simulink model "ABS_Bosch_09st"  (R2023a)
settings: Solver=ode45  StartTime=0  StopTime=20  FixedStep=0.001  RelTol=1e-3  AbsTol=1e-6
undefined symbols (not defined in the file or in its folder): DiscIntNeverNeededParam
libraries: simulink x18, dspsigops x4, Solver_SF x1
settings Model: ExtModeTrigMode=oneshot  Creator=jhu  LastModifiedBy=USER
settings SolverCC: AutoScaleAbsTol=off  AlgebraicLoopSolver=TrustRegion
settings DataIOCC: SaveFormat=Array  SignalLoggingSaveFormat=ModelDataLogs  ReturnWorkspaceOutputs=off  SignalLoggingName=sigsOut
settings OptimizationCC: BlockReduction=off  BooleanDataType=off  ExpressionDepthLimit=2147483647  LifeSpan=inf
settings DebuggingCC: SaveWithParameterizedLinksMsg=none  UnderspecifiedInitializationDetection=Classic  MergeDetectMultiDrivingBlocksExec=none  SignalResolutionControl=TryResolveAllWithWarning  MultiTaskDSMMsg=warning  MultiTaskCondExecSysMsg=none  FcnCallInpInsideContextMsg=warning  UnconnectedInputMsg=warning  UnconnectedOutputMsg=warning  UnconnectedLineMsg=warning  StateNameClashWarn=warning  SFUnexpectedBacktrackingDiag=warning  SFNoUnconditionalDefaultTransitionDiag=warning  SFExecutionAtInitializationDiag=none  ArithmeticOperatorsInVariantConditions=warning
settings HardwareCC: ProdBitPerPointer=32  ProdBitPerSizeT=32  ProdBitPerPtrDiffT=32  ProdLargestAtomicFloat=None  ProdIntDivRoundTo=Undefined  ProdEndianess=Unspecified  ProdWordSize=32  ProdHWDeviceType=32-bit Generic  TargetUnknown=on
settings ModelReferenceCC: PropagateSignalLabelsOutOfModel=off
settings SFSimCC: SimUseLocalCustomCode=off  CustomCodeUndefinedFunction=UseInterfaceOnly
settings RTWCC: TemplateMakefile=grt_vc.tmf  RTWUseLocalCustomCode=off
settings CodeAppCC: StateflowObjectComments=on
settings GRTTargetCC: TargetFcnLib=ansi_tfl_tmw.mat  TargetLangStandard=C89/C90 (ANSI)  CombineOutputUpdateFcns=off  GRTInterface=on
settings ConfigComp: CovMetricSettings=dw  CovSaveCumulativeToWorkspaceVar=on  CovSaveSingleToWorkspaceVar=on  CovExternalEMLEnable=off

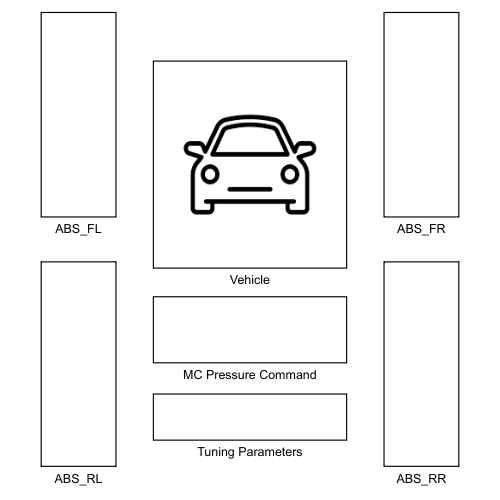
[thumbnail: Simulink's stored preview of the top-level diagram]
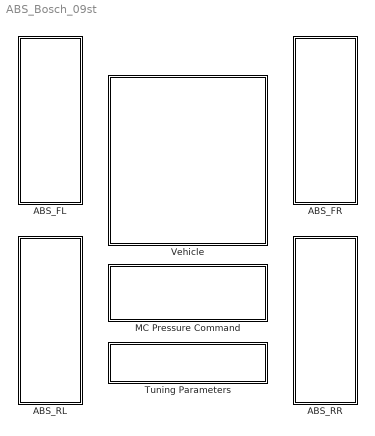
== system ABS_Bosch_09st ==
  ABS_FL : Subsystem
  ABS_FR : Subsystem
  ABS_RL : Subsystem
  ABS_RR : Subsystem
  MC Pressure Command : Subsystem
  Tuning Parameters : Subsystem
  Vehicle : Subsystem
      mask Display: image('C:\Users\USER\Downloads\vehicle_icon.png'); % Use "Edit Image" on toolstrip to change.

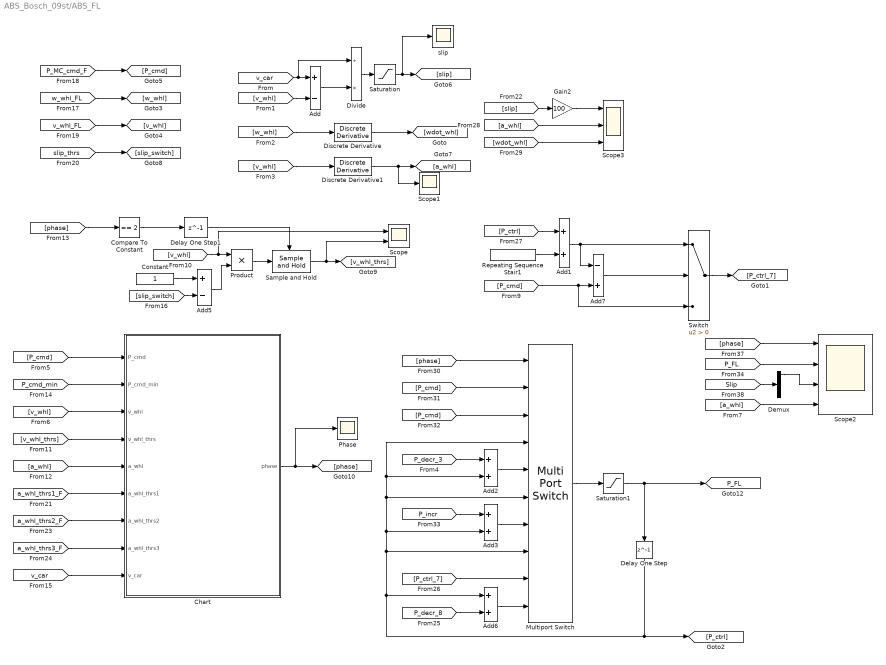
== system ABS_Bosch_09st/ABS_FL ==
  Add : Sum  Inputs=+-
  Add{1..3,6} (4 alike) : Sum
  Add5 : Sum  Inputs=+-
  Add7 : Sum  Inputs=-+
  Chart : Stateflow chart  TreatAsAtomicUnit=on
      settings: PortSchema="{\"entries\":[{\"content\":{\"sides\":[{\"content\":{\"connectorIds\":[\"In4\",\"In5\",\"In2\",\"In9\",\"In1\",\"In6\",\"In7\",\"In8\",\"In3\"]},\"type\":\"ConnectorPlacement.EquallySpacedRectSide\",\"uuid\":\"d1b40d47-5080-4bdb-9b64-2db0b8a6d570\"},{\"content\":{\"connectorIds\":[\"Out1\"],\"side\":\"RIGHT\"},\"type\":\"ConnectorPlacement.EquallySpacedRectSide\",\"uuid\":\"3562d231-244b-4945-a90c-51a654d62f0f\"},{\"content\":{\"side\":\"TOP\"},\"type\":\"ConnectorPlacement.EquallySpacedRectSide\",\"uuid\":\"6c914ffe-04dc-4ab2-bade-76d69248353c\"}]},\"type\":\"ConnectorPlacement.EquallySpacedConnector\",\"uuid\":\"36a59ec9-6bc3-461d-a020-c1da85e3b47f\"}],\"packageUris\":[\"http://schema.mathworks.com/mf0/Connector/R2020b\"],\"version\":\"1.0\"}"
  Compare To Constant : simulink/Logic and Bit Operations/Compare To Constant  relop===  const=2  OutDataTypeStr=boolean
  Constant : Constant
  Delay One Step : Delay  DelayLength=1  SampleTime=0.01
  Delay One Step1 : Delay  DelayLength=1  SampleTime=0.01
  Demux : Demux
  Discrete Derivative : simulink/Discrete/Discrete Derivative  gainval=1.0  ICPrevScaledInput=0.0  OutMin=[]  OutMax=[]  OutDataType=fixdt(1, 16)  OutScaling=2^-10  DoSatur=off
  Discrete Derivative1 : simulink/Discrete/Discrete Derivative  gainval=1.0  ICPrevScaledInput=0.0  OutMin=[]  OutMax=[]  OutDataType=fixdt(1, 16)  OutScaling=2^-10  DoSatur=off
  Divide : Product  Inputs=/*
  Gain2 : Gain  Gain=100
  Multiport Switch : MultiPortSwitch  DataPortOrder=Zero-based contiguous  Inputs=9  zeroidx=on  SaturateOnIntegerOverflow=off  InputSameDT=off
  Phase : Scope
  Product : Product
  Repeating Sequence Stair1 : simulink/Sources/Repeating Sequence Stair  OutValues=[0.2 0].'  tsamp=0.01  OutMin=[]  OutMax=[]  OutDataTypeStr=double  OutputDataTypeScalingMode=double  OutDataType=fixdt(0,8)  ConRadixGroup=Best Precision: Vector-wise  OutScaling=2^-12
  Sample and Hold : dspsigops/Sample and Hold  trig=Rising edge  initCond=0  latchinput=off
  Saturation : Saturate  UpperLimit=1  LowerLimit=-1
  Saturation1 : Saturate  UpperLimit=6  LowerLimit=0
  Scope : Scope  NumInputPorts=2
  Scope1 : Scope
  Scope2 : Scope  NumInputPorts=4
  Scope3 : Scope  NumInputPorts=3
  Switch : Switch  Criteria=u2 > Threshold  SaturateOnIntegerOverflow=off  InputSameDT=off
  slip : Scope
  tag scope: P_FL=global
  wires:
  Delay One Step/1 -> [P_ctrl], Add6/1, Multiport Switch/6, Add2/2, Multiport Switch/4, Add3/2, Multiport Switch/8
  Switch/1 -> [P_ctrl_7]
  Add7/1 -> Switch/2
  [P_cmd] -> Add7/2, Switch/3
  Add1/1 -> Add7/1, Switch/1
  Repeating Sequence Stair1/1 -> Add1/2
  [P_ctrl] -> Add1/1
  [v_car] -> Divide/1, Add/1
  [v_whl] -> Add/2
  Add/1 -> Divide/2
  Divide/1 -> Saturation/1
  Saturation/1 -> slip/1, [slip]
  [w_whl] -> Discrete Derivative/1
  Discrete Derivative/1 -> [wdot_whl]
  [v_whl] -> Discrete Derivative1/1
  Discrete Derivative1/1 -> Scope1/1, [a_whl]
  [slip_thrs] -> [slip_switch]
  [v_whl] -> Scope/1, Product/1
  Sample and Hold/1 -> Scope/2, [v_whl_thrs]
  Chart/1(phase) -> Phase/1, [phase]
  [w_whl_FL] -> [w_whl]
  [v_whl_FL] -> [v_whl]
  [P_MC_cmd_F] -> [P_cmd]
  [slip] -> Gain2/1
  [a_whl] -> Scope3/2
  [wdot_whl] -> Scope3/3
  Gain2/1 -> Scope3/1
  [phase] -> Multiport Switch/1
  [P_cmd] -> Multiport Switch/2
  [P_cmd] -> Multiport Switch/3
  Multiport Switch/1 -> Saturation1/1
  Add2/1 -> Multiport Switch/5
  [P_decr_3] -> Add2/1
  Add3/1 -> Multiport Switch/7
  [P_ctrl_7] -> Multiport Switch/9
  Saturation1/1 -> Delay One Step/1, [P_FL]
  [P_incr] -> Add3/1
  Constant/1 -> Add5/1
  [slip_switch] -> Add5/2
  Add5/1 -> Product/2
  Product/1 -> Sample and Hold/1
  [phase] -> Scope2/1
  [P_FL] -> Scope2/2
  [P_cmd] -> Chart/4(P_cmd)
  [P_cmd_min] -> Chart/5(P_cmd_min)
  [v_whl] -> Chart/2(v_whl)
  [v_whl_thrs] -> Chart/9(v_whl_thrs)
  [a_whl] -> Chart/1(a_whl)
  [v_car] -> Chart/3(v_car)
  [a_whl] -> Scope2/4
  [phase] -> Compare To Constant/1
  Compare To Constant/1 -> Delay One Step1/1
  Delay One Step1/1 -> Sample and Hold/Trigger
  [a_whl_thrs1_F] -> Chart/6(a_whl_thrs1)
  [a_whl_thrs2_F] -> Chart/7(a_whl_thrs2)
  [a_whl_thrs3_F] -> Chart/8(a_whl_thrs3)
  Add6/1 -> Multiport Switch/10
  [P_decr_8] -> Add6/2
  [Slip] -> Demux/1
  Demux/1 -> Scope2/3

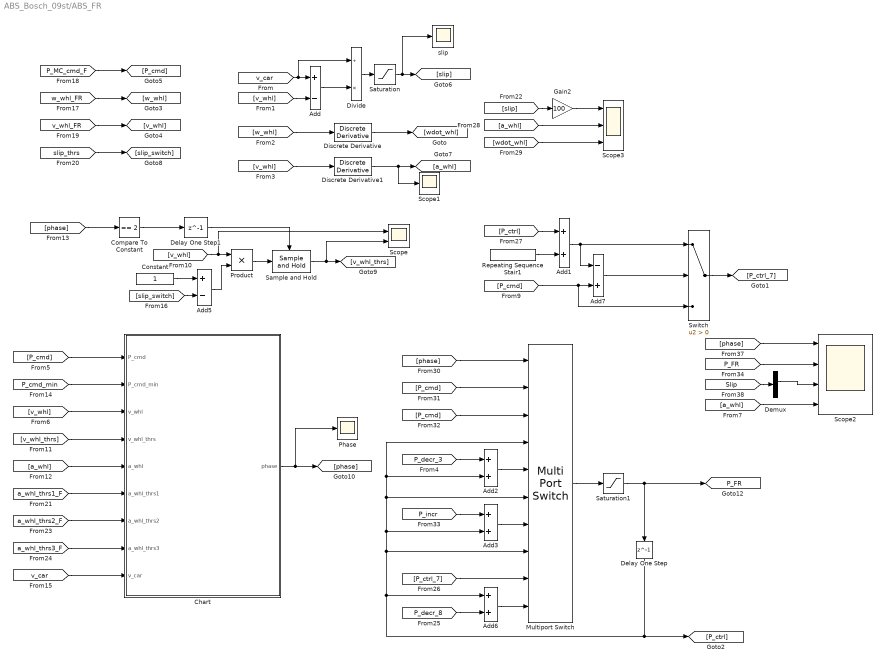
== system ABS_Bosch_09st/ABS_FR ==
  Add : Sum  Inputs=+-
  Add{1..3,6} (4 alike) : Sum
  Add5 : Sum  Inputs=+-
  Add7 : Sum  Inputs=-+
  Chart : Stateflow chart  TreatAsAtomicUnit=on
      settings: PortSchema="{\"entries\":[{\"content\":{\"sides\":[{\"content\":{\"connectorIds\":[\"In4\",\"In5\",\"In2\",\"In9\",\"In1\",\"In6\",\"In7\",\"In8\",\"In3\"]},\"type\":\"ConnectorPlacement.EquallySpacedRectSide\",\"uuid\":\"d1b40d47-5080-4bdb-9b64-2db0b8a6d570\"},{\"content\":{\"connectorIds\":[\"Out1\"],\"side\":\"RIGHT\"},\"type\":\"ConnectorPlacement.EquallySpacedRectSide\",\"uuid\":\"3562d231-244b-4945-a90c-51a654d62f0f\"},{\"content\":{\"side\":\"TOP\"},\"type\":\"ConnectorPlacement.EquallySpacedRectSide\",\"uuid\":\"6c914ffe-04dc-4ab2-bade-76d69248353c\"}]},\"type\":\"ConnectorPlacement.EquallySpacedConnector\",\"uuid\":\"36a59ec9-6bc3-461d-a020-c1da85e3b47f\"}],\"packageUris\":[\"http://schema.mathworks.com/mf0/Connector/R2020b\"],\"version\":\"1.0\"}"
  Compare To Constant : simulink/Logic and Bit Operations/Compare To Constant  relop===  const=2  OutDataTypeStr=boolean
  Constant : Constant
  Delay One Step : Delay  DelayLength=1  SampleTime=0.01
  Delay One Step1 : Delay  DelayLength=1  SampleTime=0.01
  Demux : Demux
  Discrete Derivative : simulink/Discrete/Discrete Derivative  gainval=1.0  ICPrevScaledInput=0.0  OutMin=[]  OutMax=[]  OutDataType=fixdt(1, 16)  OutScaling=2^-10  DoSatur=off
  Discrete Derivative1 : simulink/Discrete/Discrete Derivative  gainval=1.0  ICPrevScaledInput=0.0  OutMin=[]  OutMax=[]  OutDataType=fixdt(1, 16)  OutScaling=2^-10  DoSatur=off
  Divide : Product  Inputs=/*
  Gain2 : Gain  Gain=100
  Multiport Switch : MultiPortSwitch  DataPortOrder=Zero-based contiguous  Inputs=9  zeroidx=on  SaturateOnIntegerOverflow=off  InputSameDT=off
  Phase : Scope
  Product : Product
  Repeating Sequence Stair1 : simulink/Sources/Repeating Sequence Stair  OutValues=[0.2 0].'  tsamp=0.01  OutMin=[]  OutMax=[]  OutDataTypeStr=double  OutputDataTypeScalingMode=double  OutDataType=fixdt(0,8)  ConRadixGroup=Best Precision: Vector-wise  OutScaling=2^-12
  Sample and Hold : dspsigops/Sample and Hold  trig=Rising edge  initCond=0  latchinput=off
  Saturation : Saturate  UpperLimit=1  LowerLimit=-1
  Saturation1 : Saturate  UpperLimit=6  LowerLimit=0
  Scope : Scope  NumInputPorts=2
  Scope1 : Scope
  Scope2 : Scope  NumInputPorts=4
  Scope3 : Scope  NumInputPorts=3
  Switch : Switch  Criteria=u2 > Threshold  SaturateOnIntegerOverflow=off  InputSameDT=off
  slip : Scope
  tag scope: P_FR=global
  wires:
  [P_decr_8] -> Add6/2
  Add6/1 -> Multiport Switch/10
  [a_whl_thrs3_F] -> Chart/8(a_whl_thrs3)
  [a_whl_thrs2_F] -> Chart/7(a_whl_thrs2)
  [a_whl_thrs1_F] -> Chart/6(a_whl_thrs1)
  Delay One Step1/1 -> Sample and Hold/Trigger
  Compare To Constant/1 -> Delay One Step1/1
  [phase] -> Compare To Constant/1
  [a_whl] -> Scope2/4
  [v_car] -> Chart/3(v_car)
  [a_whl] -> Chart/1(a_whl)
  [v_whl_thrs] -> Chart/9(v_whl_thrs)
  [v_whl] -> Chart/2(v_whl)
  [P_cmd_min] -> Chart/5(P_cmd_min)
  [P_cmd] -> Chart/4(P_cmd)
  [Slip] -> Demux/1
  [P_FR] -> Scope2/2
  [phase] -> Scope2/1
  Product/1 -> Sample and Hold/1
  Add5/1 -> Product/2
  [slip_switch] -> Add5/2
  Constant/1 -> Add5/1
  [P_incr] -> Add3/1
  Saturation1/1 -> [P_FR], Delay One Step/1
  [P_ctrl_7] -> Multiport Switch/9
  Add3/1 -> Multiport Switch/7
  [P_decr_3] -> Add2/1
  Add2/1 -> Multiport Switch/5
  Multiport Switch/1 -> Saturation1/1
  [P_cmd] -> Multiport Switch/3
  [P_cmd] -> Multiport Switch/2
  [phase] -> Multiport Switch/1
  Gain2/1 -> Scope3/1
  [wdot_whl] -> Scope3/3
  [a_whl] -> Scope3/2
  [slip] -> Gain2/1
  [P_MC_cmd_F] -> [P_cmd]
  [v_whl_FR] -> [v_whl]
  [w_whl_FR] -> [w_whl]
  Chart/1(phase) -> [phase], Phase/1
  Sample and Hold/1 -> [v_whl_thrs], Scope/2
  [v_whl] -> Product/1, Scope/1
  [slip_thrs] -> [slip_switch]
  Discrete Derivative1/1 -> [a_whl], Scope1/1
  [v_whl] -> Discrete Derivative1/1
  Discrete Derivative/1 -> [wdot_whl]
  [w_whl] -> Discrete Derivative/1
  Saturation/1 -> [slip], slip/1
  Divide/1 -> Saturation/1
  Add/1 -> Divide/2
  [v_whl] -> Add/2
  [v_car] -> Add/1, Divide/1
  [P_ctrl] -> Add1/1
  Repeating Sequence Stair1/1 -> Add1/2
  Add1/1 -> Switch/1, Add7/1
  [P_cmd] -> Switch/3, Add7/2
  Add7/1 -> Switch/2
  Switch/1 -> [P_ctrl_7]
  Delay One Step/1 -> Multiport Switch/8, Add3/2, Multiport Switch/6, Multiport Switch/4, Add2/2, Add6/1, [P_ctrl]
  Demux/2 -> Scope2/3

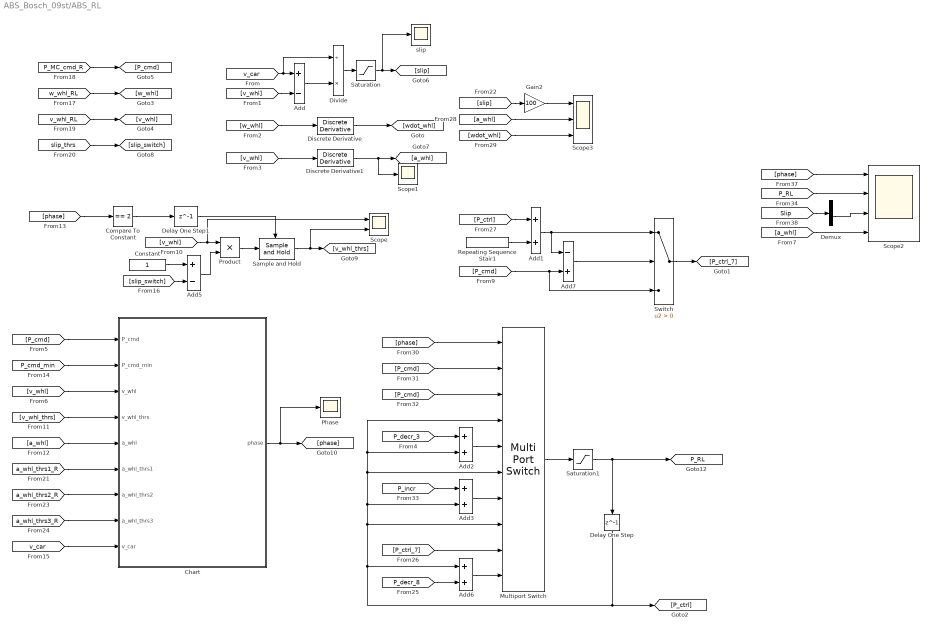
== system ABS_Bosch_09st/ABS_RL ==
  Add : Sum  Inputs=+-
  Add{1..3,6} (4 alike) : Sum
  Add5 : Sum  Inputs=+-
  Add7 : Sum  Inputs=-+
  Chart : Stateflow chart  TreatAsAtomicUnit=on
      settings: PortSchema="{\"entries\":[{\"content\":{\"sides\":[{\"content\":{\"connectorIds\":[\"In4\",\"In5\",\"In2\",\"In9\",\"In1\",\"In6\",\"In7\",\"In8\",\"In3\"]},\"type\":\"ConnectorPlacement.EquallySpacedRectSide\",\"uuid\":\"d1b40d47-5080-4bdb-9b64-2db0b8a6d570\"},{\"content\":{\"connectorIds\":[\"Out1\"],\"side\":\"RIGHT\"},\"type\":\"ConnectorPlacement.EquallySpacedRectSide\",\"uuid\":\"3562d231-244b-4945-a90c-51a654d62f0f\"},{\"content\":{\"side\":\"TOP\"},\"type\":\"ConnectorPlacement.EquallySpacedRectSide\",\"uuid\":\"6c914ffe-04dc-4ab2-bade-76d69248353c\"}]},\"type\":\"ConnectorPlacement.EquallySpacedConnector\",\"uuid\":\"36a59ec9-6bc3-461d-a020-c1da85e3b47f\"}],\"packageUris\":[\"http://schema.mathworks.com/mf0/Connector/R2020b\"],\"version\":\"1.0\"}"
  Compare To Constant : simulink/Logic and Bit Operations/Compare To Constant  relop===  const=2  OutDataTypeStr=boolean
  Constant : Constant
  Delay One Step : Delay  DelayLength=1  SampleTime=0.01
  Delay One Step1 : Delay  DelayLength=1  SampleTime=0.01
  Demux : Demux
  Discrete Derivative : simulink/Discrete/Discrete Derivative  gainval=1.0  ICPrevScaledInput=0.0  OutMin=[]  OutMax=[]  OutDataType=fixdt(1, 16)  OutScaling=2^-10  DoSatur=off
  Discrete Derivative1 : simulink/Discrete/Discrete Derivative  gainval=1.0  ICPrevScaledInput=0.0  OutMin=[]  OutMax=[]  OutDataType=fixdt(1, 16)  OutScaling=2^-10  DoSatur=off
  Divide : Product  Inputs=/*
  Gain2 : Gain  Gain=100
  Multiport Switch : MultiPortSwitch  DataPortOrder=Zero-based contiguous  Inputs=9  zeroidx=on  SaturateOnIntegerOverflow=off  InputSameDT=off
  Phase : Scope
  Product : Product
  Repeating Sequence Stair1 : simulink/Sources/Repeating Sequence Stair  OutValues=[0.2 0].'  tsamp=0.01  OutMin=[]  OutMax=[]  OutDataTypeStr=double  OutputDataTypeScalingMode=double  OutDataType=fixdt(0,8)  ConRadixGroup=Best Precision: Vector-wise  OutScaling=2^-12
  Sample and Hold : dspsigops/Sample and Hold  trig=Rising edge  initCond=0  latchinput=off
  Saturation : Saturate  UpperLimit=1  LowerLimit=-1
  Saturation1 : Saturate  UpperLimit=5  LowerLimit=0
  Scope : Scope  NumInputPorts=2
  Scope1 : Scope
  Scope2 : Scope  NumInputPorts=4
  Scope3 : Scope  NumInputPorts=3
  Switch : Switch  Criteria=u2 > Threshold  SaturateOnIntegerOverflow=off  InputSameDT=off
  slip : Scope
  tag scope: P_RL=global
  wires:
  Delay One Step/1 -> [P_ctrl], Add6/1, Multiport Switch/6, Add2/2, Multiport Switch/4, Add3/2, Multiport Switch/8
  Switch/1 -> [P_ctrl_7]
  Add7/1 -> Switch/2
  [P_cmd] -> Add7/2, Switch/3
  Add1/1 -> Add7/1, Switch/1
  Repeating Sequence Stair1/1 -> Add1/2
  [P_ctrl] -> Add1/1
  [v_car] -> Divide/1, Add/1
  [v_whl] -> Add/2
  Add/1 -> Divide/2
  Divide/1 -> Saturation/1
  Saturation/1 -> slip/1, [slip]
  [w_whl] -> Discrete Derivative/1
  Discrete Derivative/1 -> [wdot_whl]
  [v_whl] -> Discrete Derivative1/1
  Discrete Derivative1/1 -> Scope1/1, [a_whl]
  [slip_thrs] -> [slip_switch]
  [v_whl] -> Scope/1, Product/1
  Sample and Hold/1 -> Scope/2, [v_whl_thrs]
  Chart/1(phase) -> Phase/1, [phase]
  [w_whl_RL] -> [w_whl]
  [v_whl_RL] -> [v_whl]
  [P_MC_cmd_R] -> [P_cmd]
  [slip] -> Gain2/1
  [a_whl] -> Scope3/2
  [wdot_whl] -> Scope3/3
  Gain2/1 -> Scope3/1
  [phase] -> Multiport Switch/1
  [P_cmd] -> Multiport Switch/2
  [P_cmd] -> Multiport Switch/3
  Multiport Switch/1 -> Saturation1/1
  Add2/1 -> Multiport Switch/5
  [P_decr_3] -> Add2/1
  Add3/1 -> Multiport Switch/7
  [P_ctrl_7] -> Multiport Switch/9
  Saturation1/1 -> Delay One Step/1, [P_RL]
  [P_incr] -> Add3/1
  Constant/1 -> Add5/1
  [slip_switch] -> Add5/2
  Add5/1 -> Product/2
  Product/1 -> Sample and Hold/1
  [phase] -> Scope2/1
  [P_RL] -> Scope2/2
  [P_cmd] -> Chart/4(P_cmd)
  [P_cmd_min] -> Chart/5(P_cmd_min)
  [v_whl] -> Chart/2(v_whl)
  [v_whl_thrs] -> Chart/9(v_whl_thrs)
  [a_whl] -> Chart/1(a_whl)
  [v_car] -> Chart/3(v_car)
  [a_whl] -> Scope2/4
  [phase] -> Compare To Constant/1
  Compare To Constant/1 -> Delay One Step1/1
  Delay One Step1/1 -> Sample and Hold/Trigger
  [a_whl_thrs1_R] -> Chart/6(a_whl_thrs1)
  [a_whl_thrs2_R] -> Chart/7(a_whl_thrs2)
  [a_whl_thrs3_R] -> Chart/8(a_whl_thrs3)
  Add6/1 -> Multiport Switch/10
  [P_decr_8] -> Add6/2
  [Slip] -> Demux/1
  Demux/3 -> Scope2/3

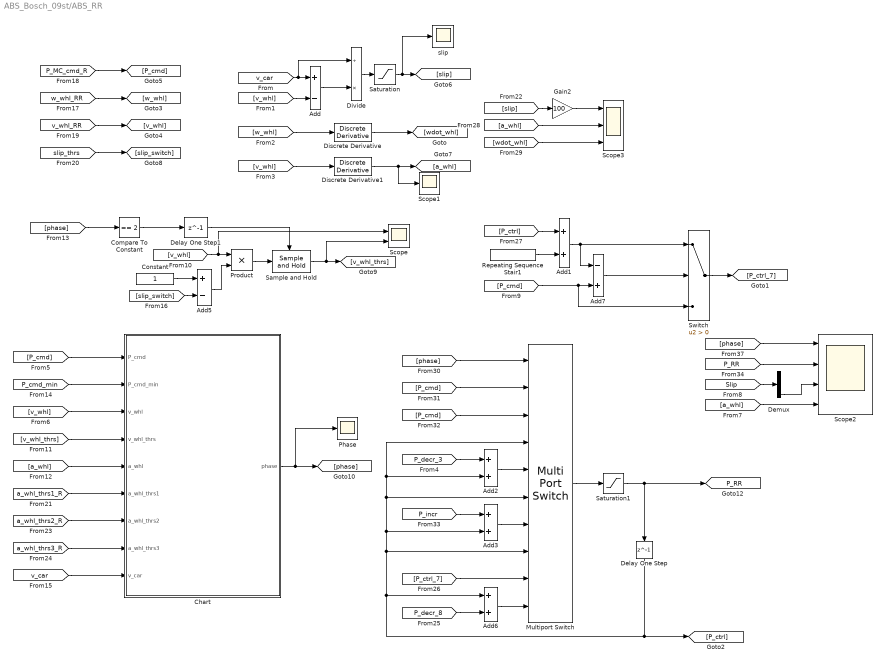
== system ABS_Bosch_09st/ABS_RR ==
  Add : Sum  Inputs=+-
  Add{1..3,6} (4 alike) : Sum
  Add5 : Sum  Inputs=+-
  Add7 : Sum  Inputs=-+
  Chart : Stateflow chart  TreatAsAtomicUnit=on
      settings: PortSchema="{\"entries\":[{\"content\":{\"sides\":[{\"content\":{\"connectorIds\":[\"In4\",\"In5\",\"In2\",\"In9\",\"In1\",\"In6\",\"In7\",\"In8\",\"In3\"]},\"type\":\"ConnectorPlacement.EquallySpacedRectSide\",\"uuid\":\"d1b40d47-5080-4bdb-9b64-2db0b8a6d570\"},{\"content\":{\"connectorIds\":[\"Out1\"],\"side\":\"RIGHT\"},\"type\":\"ConnectorPlacement.EquallySpacedRectSide\",\"uuid\":\"3562d231-244b-4945-a90c-51a654d62f0f\"},{\"content\":{\"side\":\"TOP\"},\"type\":\"ConnectorPlacement.EquallySpacedRectSide\",\"uuid\":\"6c914ffe-04dc-4ab2-bade-76d69248353c\"}]},\"type\":\"ConnectorPlacement.EquallySpacedConnector\",\"uuid\":\"36a59ec9-6bc3-461d-a020-c1da85e3b47f\"}],\"packageUris\":[\"http://schema.mathworks.com/mf0/Connector/R2020b\"],\"version\":\"1.0\"}"
  Compare To Constant : simulink/Logic and Bit Operations/Compare To Constant  relop===  const=2  OutDataTypeStr=boolean
  Constant : Constant
  Delay One Step : Delay  DelayLength=1  SampleTime=0.01
  Delay One Step1 : Delay  DelayLength=1  SampleTime=0.01
  Demux : Demux
  Discrete Derivative : simulink/Discrete/Discrete Derivative  gainval=1.0  ICPrevScaledInput=0.0  OutMin=[]  OutMax=[]  OutDataType=fixdt(1, 16)  OutScaling=2^-10  DoSatur=off
  Discrete Derivative1 : simulink/Discrete/Discrete Derivative  gainval=1.0  ICPrevScaledInput=0.0  OutMin=[]  OutMax=[]  OutDataType=fixdt(1, 16)  OutScaling=2^-10  DoSatur=off
  Divide : Product  Inputs=/*
  Gain2 : Gain  Gain=100
  Multiport Switch : MultiPortSwitch  DataPortOrder=Zero-based contiguous  Inputs=9  zeroidx=on  SaturateOnIntegerOverflow=off  InputSameDT=off
  Phase : Scope
  Product : Product
  Repeating Sequence Stair1 : simulink/Sources/Repeating Sequence Stair  OutValues=[0.2 0].'  tsamp=0.01  OutMin=[]  OutMax=[]  OutDataTypeStr=double  OutputDataTypeScalingMode=double  OutDataType=fixdt(0,8)  ConRadixGroup=Best Precision: Vector-wise  OutScaling=2^-12
  Sample and Hold : dspsigops/Sample and Hold  trig=Rising edge  initCond=0  latchinput=off
  Saturation : Saturate  UpperLimit=1  LowerLimit=-1
  Saturation1 : Saturate  UpperLimit=5  LowerLimit=0
  Scope : Scope  NumInputPorts=2
  Scope1 : Scope
  Scope2 : Scope  NumInputPorts=4
  Scope3 : Scope  NumInputPorts=3
  Switch : Switch  Criteria=u2 > Threshold  SaturateOnIntegerOverflow=off  InputSameDT=off
  slip : Scope
  tag scope: P_RR=global
  wires:
  Delay One Step/1 -> [P_ctrl], Add6/1, Multiport Switch/6, Add2/2, Multiport Switch/4, Add3/2, Multiport Switch/8
  Switch/1 -> [P_ctrl_7]
  Add7/1 -> Switch/2
  [P_cmd] -> Add7/2, Switch/3
  Add1/1 -> Add7/1, Switch/1
  Repeating Sequence Stair1/1 -> Add1/2
  [P_ctrl] -> Add1/1
  [v_car] -> Divide/1, Add/1
  [v_whl] -> Add/2
  Add/1 -> Divide/2
  Divide/1 -> Saturation/1
  Saturation/1 -> slip/1, [slip]
  [w_whl] -> Discrete Derivative/1
  Discrete Derivative/1 -> [wdot_whl]
  [v_whl] -> Discrete Derivative1/1
  Discrete Derivative1/1 -> Scope1/1, [a_whl]
  [slip_thrs] -> [slip_switch]
  [v_whl] -> Scope/1, Product/1
  Sample and Hold/1 -> Scope/2, [v_whl_thrs]
  Chart/1(phase) -> Phase/1, [phase]
  [w_whl_RR] -> [w_whl]
  [v_whl_RR] -> [v_whl]
  [P_MC_cmd_R] -> [P_cmd]
  [slip] -> Gain2/1
  [a_whl] -> Scope3/2
  [wdot_whl] -> Scope3/3
  Gain2/1 -> Scope3/1
  [phase] -> Multiport Switch/1
  [P_cmd] -> Multiport Switch/2
  [P_cmd] -> Multiport Switch/3
  Multiport Switch/1 -> Saturation1/1
  Add2/1 -> Multiport Switch/5
  [P_decr_3] -> Add2/1
  Add3/1 -> Multiport Switch/7
  [P_ctrl_7] -> Multiport Switch/9
  Saturation1/1 -> Delay One Step/1, [P_RR]
  [P_incr] -> Add3/1
  Constant/1 -> Add5/1
  [slip_switch] -> Add5/2
  Add5/1 -> Product/2
  Product/1 -> Sample and Hold/1
  [phase] -> Scope2/1
  [P_RR] -> Scope2/2
  [P_cmd] -> Chart/4(P_cmd)
  [P_cmd_min] -> Chart/5(P_cmd_min)
  [v_whl] -> Chart/2(v_whl)
  [v_whl_thrs] -> Chart/9(v_whl_thrs)
  [a_whl] -> Chart/1(a_whl)
  [v_car] -> Chart/3(v_car)
  [a_whl] -> Scope2/4
  [phase] -> Compare To Constant/1
  Compare To Constant/1 -> Delay One Step1/1
  Delay One Step1/1 -> Sample and Hold/Trigger
  [a_whl_thrs1_R] -> Chart/6(a_whl_thrs1)
  [a_whl_thrs2_R] -> Chart/7(a_whl_thrs2)
  [a_whl_thrs3_R] -> Chart/8(a_whl_thrs3)
  Add6/1 -> Multiport Switch/10
  [P_decr_8] -> Add6/2
  Demux/4 -> Scope2/3
  [Slip] -> Demux/1

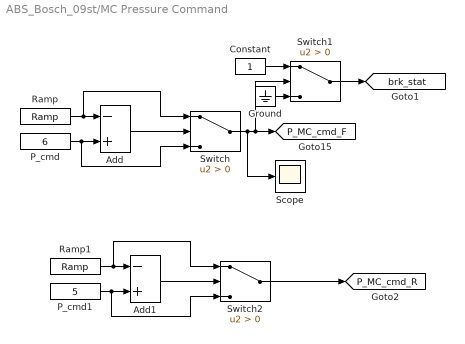
== system ABS_Bosch_09st/MC Pressure Command ==
  Add : Sum  Inputs=-+
  Add1 : Sum  Inputs=-+
  Constant : Constant
  Ground : Ground
  P_cmd : Constant  Value=6  SampleTime=0.01
  P_cmd1 : Constant  Value=5  SampleTime=0.01
  Ramp : simulink/Sources/Ramp  slope=20  start=2  InitialOutput=0
  Ramp1 : simulink/Sources/Ramp  slope=20  start=2  InitialOutput=0
  Scope : Scope
  Switch : Switch  Criteria=u2 > Threshold  SaturateOnIntegerOverflow=off  InputSameDT=off
  Switch1 : Switch  Criteria=u2 > Threshold  SaturateOnIntegerOverflow=off  InputSameDT=off
  Switch2 : Switch  Criteria=u2 > Threshold  SaturateOnIntegerOverflow=off  InputSameDT=off
  tag scope: P_MC_cmd_F=global, P_MC_cmd_R=global, brk_stat=global
  wires:
  P_cmd/1 -> Switch/3, Add/2
  Ramp/1 -> Switch/1, Add/1
  Add/1 -> Switch/2
  Switch/1 -> Scope/1, Switch1/2, [P_MC_cmd_F]
  Constant/1 -> Switch1/1
  Ground/1 -> Switch1/3
  Switch1/1 -> [brk_stat]
  Add1/1 -> Switch2/2
  Ramp1/1 -> Switch2/1, Add1/1
  P_cmd1/1 -> Switch2/3, Add1/2
  Switch2/1 -> [P_MC_cmd_R]

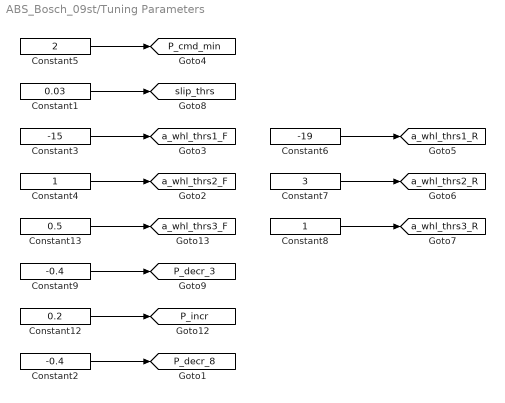
== system ABS_Bosch_09st/Tuning Parameters ==
  Constant1 : Constant  Value=0.03  SampleTime=0.01
  Constant12 : Constant  Value=0.2  SampleTime=0.01
  Constant13 : Constant  Value=0.5  SampleTime=0.01
  Constant2 : Constant  Value=-0.4  SampleTime=0.01
  Constant3 : Constant  Value=-15  SampleTime=0.01
  Constant4 : Constant  SampleTime=0.01
  Constant5 : Constant  Value=2  SampleTime=0.01
  Constant6 : Constant  Value=-19  SampleTime=0.01
  Constant7 : Constant  Value=3  SampleTime=0.01
  Constant8 : Constant  SampleTime=0.01
  Constant9 : Constant  Value=-0.4  SampleTime=0.01
  tag scope: P_cmd_min=global, P_decr_3=global, P_decr_8=global, P_incr=global, a_whl_thrs1_F=global, a_whl_thrs1_R=global, a_whl_thrs2_F=global, a_whl_thrs2_R=global, a_whl_thrs3_F=global, a_whl_thrs3_R=global, slip_thrs=global
  wires:
  Constant1/1 -> [slip_thrs]
  Constant4/1 -> [a_whl_thrs2_F]
  Constant3/1 -> [a_whl_thrs1_F]
  Constant5/1 -> [P_cmd_min]
  Constant9/1 -> [P_decr_3]
  Constant12/1 -> [P_incr]
  Constant13/1 -> [a_whl_thrs3_F]
  Constant2/1 -> [P_decr_8]
  Constant6/1 -> [a_whl_thrs1_R]
  Constant7/1 -> [a_whl_thrs2_R]
  Constant8/1 -> [a_whl_thrs3_R]

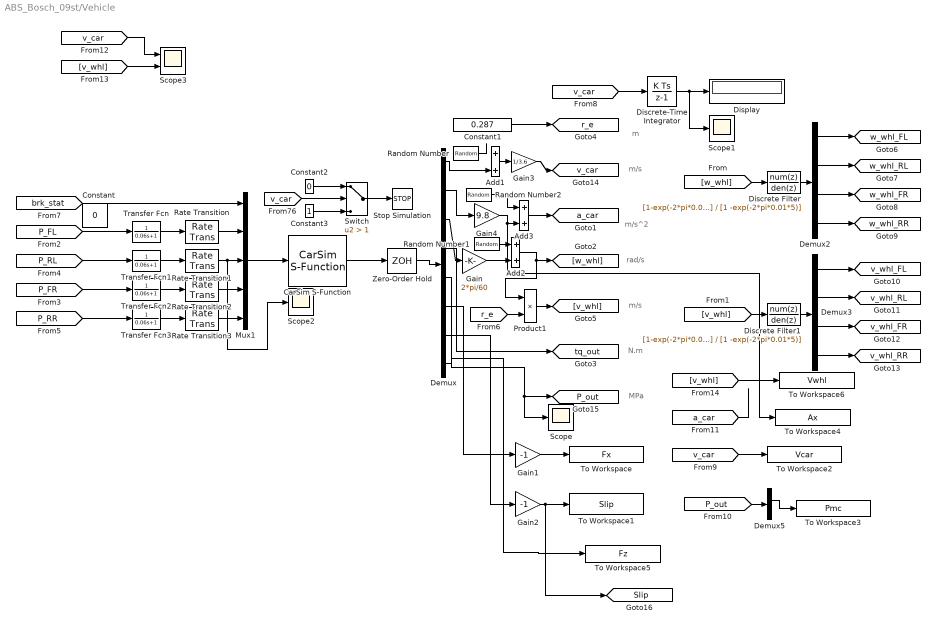
== system ABS_Bosch_09st/Vehicle ==
  note: m/s
  note: m
  note: m/s
  note: rad/s
  note: N.m
  note: m/s^2
  note: MPa
  Add1 : Sum
  Add2 : Sum
  Add3 : Sum
  CarSim S-Function : Solver_SF/CarSim S-Function  Priority=1  SIMFILE=simfile.sim  Run_RTs=off  vs_state_ind=Run  StopMode_ind=Vehicle Model
  Constant : Constant  Value=0
  Constant1 : Constant  Value=0.287
  Constant2 : Constant  Value=0
  Constant3 : Constant
  Demux : Demux  Outputs=[1 1 4 4 4 4 4 4]
  Demux2 : Demux
  Demux3 : Demux
  Demux5 : Demux
  Discrete Filter : DiscreteFilter  Numerator=[1-exp(-2*pi*0.01*5)]  Denominator=[1 -exp(-2*pi*0.01*5)]  SampleTime=0.01
  Discrete Filter1 : DiscreteFilter  Numerator=[1-exp(-2*pi*0.01*5)]  Denominator=[1 -exp(-2*pi*0.01*5)]  SampleTime=0.01
  Discrete-Time Integrator : DiscreteIntegrator  SampleTime=0.01  ICPrevOutput=DiscIntNeverNeededParam  ICPrevScaledInput=DiscIntNeverNeededParam
  Display : Display
      settings: Format=bank
  Gain : Gain  Gain=2*pi/60
  Gain1 : Gain  Gain=-1
  Gain2 : Gain  Gain=-1
  Gain3 : Gain  Gain=1/3.6
  Gain4 : Gain  Gain=9.8
  Mux1 : Mux  Inputs=5
  Product1 : Product
  Random Number : RandomNumber  Variance=0.0005  Seed=2  SampleTime=0.01
  Random Number1 : RandomNumber  Variance=0.0003  SampleTime=0.01
  Random Number2 : RandomNumber  Variance=0.001  Seed=2  SampleTime=0.01
  Rate Transition{,1..3} (4 alike) : RateTransition  OutPortSampleTime=0.01
  Scope : Scope
  Scope1 : Scope
  Scope2 : Scope
  Scope3 : Scope  NumInputPorts=2
  Stop Simulation : Stop
  Switch : Switch  Criteria=u2 > Threshold  Threshold=1  SaturateOnIntegerOverflow=off  InputSameDT=off
  To Workspace : ToWorkspace  VariableName=Fx  SaveFormat=Timeseries  SampleTime=-1
  To Workspace1 : ToWorkspace  VariableName=Slip  SaveFormat=Timeseries  SampleTime=-1
  To Workspace2 : ToWorkspace  VariableName=Vcar  SaveFormat=Timeseries  SampleTime=-1
  To Workspace3 : ToWorkspace  VariableName=Pmc  SaveFormat=Timeseries  SampleTime=-1
  To Workspace4 : ToWorkspace  VariableName=Ax  SaveFormat=Timeseries  SampleTime=-1
  To Workspace5 : ToWorkspace  VariableName=Fz  SaveFormat=Timeseries  SampleTime=-1
  To Workspace6 : ToWorkspace  VariableName=Vwhl  SaveFormat=Timeseries  SampleTime=-1
  Transfer Fcn{,1..3} (4 alike) : TransferFcn  Denominator=[0.06 1]
  Zero-Order Hold : ZeroOrderHold  SampleTime=0.01
  tag scope: P_out=global, Slip=global, a_car=global, r_e=global, tq_out=global, v_car=global, v_whl_FL=global, v_whl_FR=global, v_whl_RL=global, v_whl_RR=global, w_whl_FL=global, w_whl_FR=global, w_whl_RL=global, w_whl_RR=global
  wires:
  Constant1/1 -> [r_e]
  [r_e] -> Product1/2
  Product1/1 -> [v_whl]
  Demux3/4 -> [v_whl_RR]
  Demux3/2 -> [v_whl_RL]
  Demux3/1 -> [v_whl_FL]
  Demux3/3 -> [v_whl_FR]
  Gain/1 -> Add2/2
  Demux/3 -> Gain/1
  Gain4/1 -> To Workspace4/1, Add3/2
  Demux/4 -> [tq_out]
  CarSim S-Function/1 -> Zero-Order Hold/1
  Demux2/2 -> [w_whl_RL]
  Gain3/1 -> [v_car]
  Demux2/1 -> [w_whl_FL]
  Demux/1 -> Add1/2
  Demux2/3 -> [w_whl_FR]
  Zero-Order Hold/1 -> Demux/1
  Demux2/4 -> [w_whl_RR]
  Transfer Fcn/1 -> Rate Transition/1
  Transfer Fcn1/1 -> Rate Transition1/1
  Transfer Fcn2/1 -> Rate Transition2/1
  Transfer Fcn3/1 -> Rate Transition3/1
  Mux1/1 -> CarSim S-Function/1
  Rate Transition/1 -> Mux1/2
  Rate Transition1/1 -> Scope2/1, Mux1/3
  Rate Transition2/1 -> Mux1/4
  Rate Transition3/1 -> Mux1/5
  Demux/5 -> Scope/1, [P_out]
  [P_FR] -> Transfer Fcn2/1
  [P_RL] -> Transfer Fcn1/1
  [P_RR] -> Transfer Fcn3/1
  Demux/2 -> Gain4/1
  Random Number/1 -> ?
  Add1/1 -> Gain3/1
  Add2/1 -> Product1/1, [w_whl]
  [brk_stat] -> Mux1/1
  Random Number1/1 -> Add2/1
  [w_whl] -> Discrete Filter/1
  [v_whl] -> Discrete Filter1/1
  Discrete Filter1/1 -> Demux3/1
  Discrete Filter/1 -> Demux2/1
  [v_car] -> Switch/2
  Constant3/1 -> Switch/3
  Switch/1 -> Stop Simulation/1
  Constant2/1 -> Switch/1
  [v_car] -> Discrete-Time Integrator/1
  Discrete-Time Integrator/1 -> Scope1/1, Display/1
  Random Number2/1 -> Add3/1
  Add3/1 -> [a_car]
  Gain1/1 -> To Workspace/1
  Gain2/1 -> [Slip], To Workspace1/1
  [v_car] -> To Workspace2/1
  [P_out] -> Demux5/1
  Demux/6 -> Gain1/1
  Demux/7 -> Gain2/1
  Demux5/2 -> To Workspace3/1
  [a_car] -> ?
  Demux/8 -> To Workspace5/1
  [P_FL] -> Transfer Fcn/1
  [v_car] -> Scope3/1
  [v_whl] -> Scope3/2
  [v_whl] -> To Workspace6/1

== stateflow chart ABS_Bosch_09st/ABS_FR/Chart ==
  state ABS_On
    state Phase1
      entry,during:
      phase = 1;
    state Phase2
      entry,during:
      phase = 2;
    state Phase3
      entry,during:
      phase = 3;
    state Phase4
      entry,during:
      phase = 4;
    state Phase5
      entry,during:
      phase = 5;
    state Phase6
      entry,during:
      phase = 6;
    state Phase7
      entry,during:
      phase = 7;
    state Phase8
      entry,during:
      phase = 8;
    (default) -> Phase1
    Phase1 -> Phase2 : [(a_whl<a_whl_thrs1)]
    Phase2 -> Phase3 : [(v_whl<v_whl_thrs)]
    Phase3 -> Phase4 : [(a_whl>a_whl_thrs1)]
    (junction 81) -> Phase4
    (junction 79) -> (junction 81)
    Phase4 -> Phase5 : [(a_whl>a_whl_thrs2)]
    Phase5 -> Phase6 : [(a_whl<a_whl_thrs2)]
    Phase6 -> Phase7 : [(a_whl<a_whl_thrs3)]
    Phase7 -> Phase8 : [(a_whl<a_whl_thrs1)]
    Phase8 -> (junction 79) : [(a_whl>a_whl_thrs1)]
  state ABS_Off
    phase = 0;
  (default) -> ABS_Off
  ABS_Off -> ABS_On : [(P_cmd > P_cmd_min)&(v_car > 2)]
  (junction 96) -> ABS_Off
  ABS_On -> (junction 96) : [(P_cmd < P_cmd_min)|(v_car < 2)]
  data: a_whl input; phase output; v_whl input; v_car input; P_cmd input; P_cmd_min input; a_whl_thrs1 input; a_whl_thrs2 input; a_whl_thrs3 input; v_whl_thrs input

== stateflow chart ABS_Bosch_09st/ABS_FL/Chart ==
  state ABS_On
    state Phase1
      entry,during:
      phase = 1;
    state Phase2
      entry,during:
      phase = 2;
    state Phase3
      entry,during:
      phase = 3;
    state Phase4
      entry,during:
      phase = 4;
    state Phase5
      entry,during:
      phase = 5;
    state Phase6
      entry,during:
      phase = 6;
    state Phase7
      entry,during:
      phase = 7;
    state Phase8
      entry,during:
      phase = 8;
    (default) -> Phase1
    Phase1 -> Phase2 : [(a_whl<a_whl_thrs1)]
    Phase2 -> Phase3 : [(v_whl<v_whl_thrs)]
    Phase3 -> Phase4 : [(a_whl>a_whl_thrs1)]
    (junction 81) -> Phase4
    (junction 79) -> (junction 81)
    Phase4 -> Phase5 : [(a_whl>a_whl_thrs2)]
    Phase5 -> Phase6 : [(a_whl<a_whl_thrs2)]
    Phase6 -> Phase7 : [(a_whl<a_whl_thrs3)]
    Phase7 -> Phase8 : [(a_whl<a_whl_thrs1)]
    Phase8 -> (junction 79) : [(a_whl>a_whl_thrs1)]
  state ABS_Off
    phase = 0;
  (default) -> ABS_Off
  ABS_Off -> ABS_On : [(P_cmd > P_cmd_min)&(v_car > 2)]
  (junction 96) -> ABS_Off
  ABS_On -> (junction 96) : [(P_cmd < P_cmd_min)|(v_car < 2)]
  data: a_whl input; phase output; v_whl input; v_car input; P_cmd input; P_cmd_min input; a_whl_thrs1 input; a_whl_thrs2 input; a_whl_thrs3 input; v_whl_thrs input

== stateflow chart ABS_Bosch_09st/ABS_RR/Chart ==
  state ABS_On
    state Phase1
      entry,during:
      phase = 1;
    state Phase2
      entry,during:
      phase = 2;
    state Phase3
      entry,during:
      phase = 3;
    state Phase4
      entry,during:
      phase = 4;
    state Phase5
      entry,during:
      phase = 5;
    state Phase6
      entry,during:
      phase = 6;
    state Phase7
      entry,during:
      phase = 7;
    state Phase8
      entry,during:
      phase = 8;
    (default) -> Phase1
    Phase1 -> Phase2 : [(a_whl<a_whl_thrs1)]
    Phase2 -> Phase3 : [(v_whl<v_whl_thrs)]
    Phase3 -> Phase4 : [(a_whl>a_whl_thrs1)]
    (junction 81) -> Phase4
    (junction 79) -> (junction 81)
    Phase4 -> Phase5 : [(a_whl>a_whl_thrs2)]
    Phase5 -> Phase6 : [(a_whl<a_whl_thrs2)]
    Phase6 -> Phase7 : [(a_whl<a_whl_thrs3)]
    Phase7 -> Phase8 : [(a_whl<a_whl_thrs1)]
    Phase8 -> (junction 79) : [(a_whl>a_whl_thrs1)]
  state ABS_Off
    phase = 0;
  (default) -> ABS_Off
  ABS_Off -> ABS_On : [(P_cmd > P_cmd_min)&(v_car > 2)]
  (junction 96) -> ABS_Off
  ABS_On -> (junction 96) : [(P_cmd < P_cmd_min)|(v_car < 2)]
  data: a_whl input; phase output; v_whl input; v_car input; P_cmd input; P_cmd_min input; a_whl_thrs1 input; a_whl_thrs2 input; a_whl_thrs3 input; v_whl_thrs input

== stateflow chart ABS_Bosch_09st/ABS_RL/Chart ==
  state ABS_On
    state Phase1
      entry,during:
      phase = 1;
    state Phase2
      entry,during:
      phase = 2;
    state Phase3
      entry,during:
      phase = 3;
    state Phase4
      entry,during:
      phase = 4;
    state Phase5
      entry,during:
      phase = 5;
    state Phase6
      entry,during:
      phase = 6;
    state Phase7
      entry,during:
      phase = 7;
    state Phase8
      entry,during:
      phase = 8;
    (default) -> Phase1
    Phase1 -> Phase2 : [(a_whl<a_whl_thrs1)]
    Phase2 -> Phase3 : [(v_whl<v_whl_thrs)]
    Phase3 -> Phase4 : [(a_whl>a_whl_thrs1)]
    (junction 81) -> Phase4
    (junction 79) -> (junction 81)
    Phase4 -> Phase5 : [(a_whl>a_whl_thrs2)]
    Phase5 -> Phase6 : [(a_whl<a_whl_thrs2)]
    Phase6 -> Phase7 : [(a_whl<a_whl_thrs3)]
    Phase7 -> Phase8 : [(a_whl<a_whl_thrs1)]
    Phase8 -> (junction 79) : [(a_whl>a_whl_thrs1)]
  state ABS_Off
    phase = 0;
  (default) -> ABS_Off
  ABS_Off -> ABS_On : [(P_cmd > P_cmd_min)&(v_car > 2)]
  (junction 96) -> ABS_Off
  ABS_On -> (junction 96) : [(P_cmd < P_cmd_min)|(v_car < 2)]
  data: a_whl input; phase output; v_whl input; v_car input; P_cmd input; P_cmd_min input; a_whl_thrs1 input; a_whl_thrs2 input; a_whl_thrs3 input; v_whl_thrs input
